simulink model "Lab1_Linear"  (R2020b)
settings: Solver=VariableStepAuto  StartTime=0.0  StopTime=500  RelTol=1e-3
values from neighbouring files (symbols this model uses):
  a = 24    [Lab1.m]
  change = inv([1/S 1/S; (Tw - T0)/(S*H0) (Tc - T0)/(S*H0)])    [Lab1.m]
  gHSlow = inv(1*inv(a/(2*S*sqrt(H0)) + 1*kHSlow)*1)    [Lab1.m]
  gThetaSlow = inv(1*inv((2*Q0)/(S*H0) + 1*kThetaSlow)*1)    [Lab1.m]
  H0 = 16    [Lab1.m]
  kHSlow = -0.75*a/(2*S*sqrt(H0))    [Lab1.m]
  kThetaSlow = -0.75*(2*Q0)/(S*H0)    (= -0.0572957795131)    [Lab1.m]
  Q0 = 48    [Lab1.m]
  S = pi*5*5    (= 78.5398163397)    [Lab1.m]
  T0 = 45    [Lab1.m]
  Tc = 20    [Lab1.m]
  Tw = 70    [Lab1.m]
settings Model: Creator=DELL  LastModifiedBy=DELL

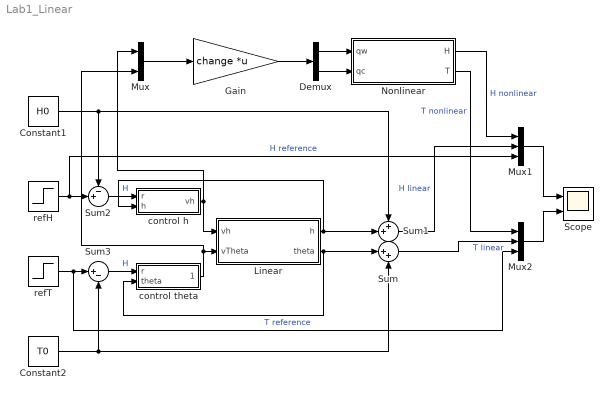
== system Lab1_Linear ==
  Constant1 : Constant  Value=H0
  Constant2 : Constant  Value=T0
  Demux : Demux  Outputs=2
  Gain : Gain  Gain=change  Multiplication=Matrix(K*u) (u vector)
  Linear : Subsystem
  Mux : Mux  Inputs=2
  Mux1 : Mux  Inputs=3
  Mux2 : Mux  Inputs=3
  Nonlinear : Subsystem
  Scope : Scope  NumInputPorts=2
  Sum : Sum  Inputs=|++
  Sum1 : Sum  Inputs=++|
  Sum2 : Sum  Inputs=-+|
  Sum3 : Sum  Inputs=|+-
  control h : Subsystem
  control theta : Subsystem
  refH : Step  Before=H0  After=17  SampleTime=0
  refT : Step  Before=T0  After=46  SampleTime=0
  wires:
  Demux/1 -> Nonlinear/1(qw)
  Demux/2 -> Nonlinear/2(qc)
  Gain/1 -> Demux/1
  Mux/1 -> Gain/1
  Mux1/1 -> Scope/1
  Nonlinear/1(H) -> Mux1/1  "H nonlinear"
  Nonlinear/2(T) -> Mux2/1  "T nonlinear"
  Mux2/1 -> Scope/2
  Linear/1(h) -> control h/2(h), Sum1/2
  Linear/2(theta) -> control theta/2(theta), Sum/1
  Sum1/1 -> Mux1/2  "H linear"
  Sum/1 -> Mux2/2  "T linear"
  Constant1/1 -> Sum1/1, Sum2/1
  Constant2/1 -> Sum3/2, Sum/2
  refH/1 -> Mux1/3, Sum2/2  "H reference"
  refT/1 -> Sum3/1, Mux2/3  "T reference"
  control theta/1(vTheta) -> Mux/2, Linear/2(vTheta)
  control h/1(vh) -> Mux/1, Linear/1(vh)
  Sum3/1 -> control theta/1(r)  "H"
  Sum2/1 -> control h/1(r)  "H"

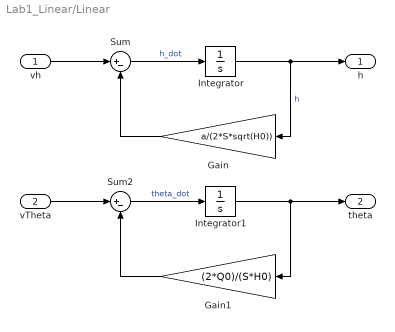
== system Lab1_Linear/Linear ==
  vh : Inport
  vTheta : Inport  Port=2
  Gain : Gain  Gain=a/(2*S*sqrt(H0))
  Gain1 : Gain  Gain=(2*Q0)/(S*H0)
  Integrator : Integrator
  Integrator1 : Integrator
  Sum : Sum  Inputs=|+-
  Sum2 : Sum  Inputs=|+-
  h : Outport
  theta : Outport  Port=2
  wires:
  vh/1 -> Sum/1
  Sum/1 -> Integrator/1  "h_dot"
  Integrator/1 -> h/1, Gain/1  "h"
  Gain/1 -> Sum/2
  Integrator1/1 -> theta/1, Gain1/1
  vTheta/1 -> Sum2/1
  Gain1/1 -> Sum2/2
  Sum2/1 -> Integrator1/1  "theta_dot"

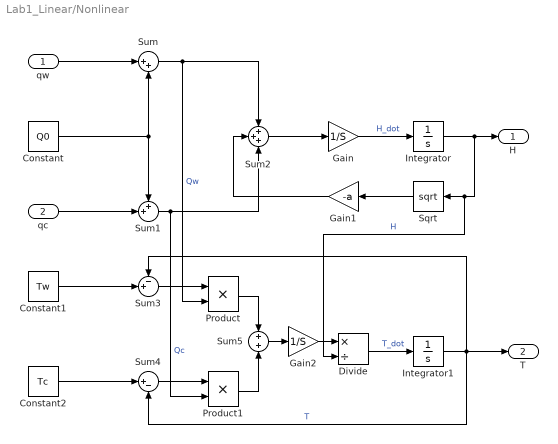
== system Lab1_Linear/Nonlinear ==
  qw : Inport
  qc : Inport  Port=2
  Constant : Constant  Value=Q0
  Constant1 : Constant  Value=Tw
  Constant2 : Constant  Value=Tc
  Divide : Product  Inputs=*/
  Gain : Gain  Gain=1/S
  Gain1 : Gain  Gain=-a
  Gain2 : Gain  Gain=1/S
  Integrator : Integrator  InitialCondition=H0
  Integrator1 : Integrator  InitialCondition=T0
  Product : Product
  Product1 : Product
  Sqrt : Sqrt  SaturateOnIntegerOverflow=on
  Sum : Sum  Inputs=|++
  Sum1 : Sum  Inputs=++|
  Sum2 : Sum  Inputs=+++
  Sum3 : Sum  Inputs=-+|
  Sum4 : Sum  Inputs=|+-
  Sum5 : Sum  Inputs=+|+
  H : Outport
  T : Outport  Port=2
  wires:
  qw/1 -> Sum/1
  Constant/1 -> Sum/2, Sum1/1
  qc/1 -> Sum1/2
  Sum/1 -> Product/2, Sum2/1  "Qw"
  Sum1/1 -> Product1/2, Sum2/3  "Qc"
  Integrator/1 -> Divide/2, Sqrt/1, H/1  "H"
  Sum2/1 -> Gain/1
  Gain/1 -> Integrator/1  "H_dot"
  Gain1/1 -> Sum2/2
  Sqrt/1 -> Gain1/1
  Integrator1/1 -> Sum4/2, T/1, Sum3/1  "T"
  Constant2/1 -> Sum4/1
  Constant1/1 -> Sum3/2
  Sum3/1 -> Product/1
  Sum4/1 -> Product1/1
  Sum5/1 -> Gain2/1
  Product/1 -> Sum5/1
  Product1/1 -> Sum5/2
  Gain2/1 -> Divide/1
  Divide/1 -> Integrator1/1  "T_dot"

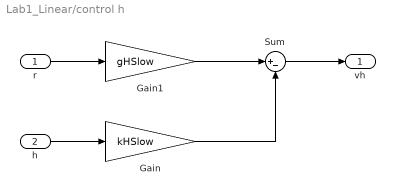
== system Lab1_Linear/control h ==
  r : Inport
  h : Inport  Port=2
  Gain : Gain  Gain=kHSlow
  Gain1 : Gain  Gain=gHSlow
  Sum : Sum  Inputs=|+-
  vh : Outport
  wires:
  r/1 -> Gain1/1
  h/1 -> Gain/1
  Gain1/1 -> Sum/1
  Gain/1 -> Sum/2
  Sum/1 -> vh/1

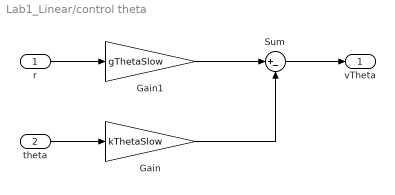
== system Lab1_Linear/control theta ==
  r : Inport
  theta : Inport  Port=2
  Gain : Gain  Gain=kThetaSlow
  Gain1 : Gain  Gain=gThetaSlow
  Sum : Sum  Inputs=|+-
  vTheta : Outport
  wires:
  r/1 -> Gain1/1
  theta/1 -> Gain/1
  Gain1/1 -> Sum/1
  Gain/1 -> Sum/2
  Sum/1 -> vTheta/1
